simulink model "Casc_Filter_reva"  (Simulink 6.6)
settings: Solver=ode45  StartTime=0.0  StopTime=32768/sampling_freq  RelTol=1e-3
values from neighbouring files (symbols this model uses):
  filter_clk = sampling_freq*clk_mult    (= 375000000)    [Cascade_Taps_reva.m]    (also in Casecade_Taps.m)
  h_g = round(h_g*2^17)/2^17    [Cascade_Taps_reva.m]    (also in Casecade_Taps.m)
  h_k = round(h_k*2^17)/2^17    [Cascade_Taps_reva.m]    (also in Casecade_Taps.m)
  sampling_freq = 125e6    (= 125000000)    [Cascade_Taps_reva.m]    (also in Casecade_Taps.m)
undefined symbols (not defined in the file or in its folder): A, B, Fs, get, PCIN
libraries: xbsIndex_r4 x314, dspsnks4 x3, dspsrcs4 x2, simulink x2
(part 2 of 3)

== system Casc_Filter_reva/DDC/DDC A/Polyphase Kaiser FIR Filter/MAC0 ==
  Count : Inport
  Data In : Inport  Port=2
  Symm Data : Inport  Port=3
  Coeff : Inport  Port=4
  Count Inv : Inport  Port=5
  ASR : xbsIndex_r4/Addressable Shift Register  infer_latency=off  depth=8  initVector=[0]  en=off  dbl_ovrd=off  use_behavioral_HDL=off  use_rpm=off  block_type=addrsr
      settings: block_version=8.2
      settings: infoedit=|
      | Delay of  configurable length.  Any element  in the delay
      |     line   can    be   addressed   and   driven    onto   the   output
      |     port.<P><P>Hardware  notes: Implemented  using SRL16s.
      |     If Virtex-4, Virtex-II or Spartan-3 devices are used, multiple SRLC16s are cascaded together.
  ASR1 : xbsIndex_r4/Addressable Shift Register  infer_latency=off  depth=8  initVector=[0]  en=off  dbl_ovrd=off  use_behavioral_HDL=off  use_rpm=off  block_type=addrsr
      settings: block_version=8.2
      settings: infoedit=|
      | Delay of  configurable length.  Any element  in the delay
      |     line   can    be   addressed   and   driven    onto   the   output
      |     port.<P><P>Hardware  notes: Implemented  using SRL16s.
      |     If Virtex-4, Virtex-II or Spartan-3 devices are used, multiple SRLC16s are cascaded together.
  AddSub1 : xbsIndex_r4/AddSub  mode=Subtraction  use_carryin=off  use_carryout=off  en=off  latency=1  precision=User Defined  arith_type="Signed  (2's comp)"  n_bits=18  bin_pt=16  quantization="Round  (unbiased: +/- Inf)"  overflow=Saturate  dbl_ovrd=off  use_behavioral_HDL=off  pipelined=on  use_rpm=on  block_type=addsub
      settings: block_version=8.2
  Constant4 : xbsIndex_r4/Constant  arith_type=DSP48 Instruction  const=5  n_bits=7  bin_pt=0  explicit_period=off  period=1  equ=P=+(A*B)  opselect=A * B  inp2=PCIN>>17  opr=+  inp1=P  carry=CIN  dbl_ovrd=off  block_type=constant
      settings: block_version=VER_STRING_GOES_HERE
  DSP1 : xbsIndex_r4/DSP48  use_b=Direct from B Port  use_op=on  use_creg=off  use_pcin=off  use_pcout=on  use_bcout=off  rst_all=off  en_all=off  pipeline_a=1  pipeline_b=1  pipeline_c=on  pipeline_p=on  pipeline_mult=on  pipeline_opmode=off  pipeline_sub=off  pipeline_carryin=off  pipeline_carryinsel=off  rst_a=off  rst_b=off  rst_c=off  rst_mult=off  rst_p=off  rst_carry_in=off  rst_ctrl=off  en_a=off  en_b=off  en_c=off  en_mult=off  en_p=off  en_carry_in=off  en_ctrl=off  dbl_ovrd=off  use_synth_model=off  xl_useadderonly=off  block_type=dsp48
      settings: block_version=8.2
  Delay : xbsIndex_r4/Delay  en=off  latency=2  dbl_ovrd=off  reg_retiming=off  block_type=delay
      settings: infoedit=Hardware notes: A delay line is a chain, each link of which is an SRL16 followed by a flip-flop. If register retiming is enabled, the delay line is a chain of flip-flops.  block_version=8.2
  Delay3 : xbsIndex_r4/Delay  en=off  latency=8  dbl_ovrd=off  reg_retiming=off  block_type=delay
      settings: infoedit=Hardware notes: A delay line is a chain, each link of which is an SRL16 followed by a flip-flop. If register retiming is enabled, the delay line is a chain of flip-flops.  block_version=8.2
  Register : xbsIndex_r4/Register  init=0  rst=off  en=off  dbl_ovrd=off  block_type=register
      settings: block_version=8.2
  Register1 : xbsIndex_r4/Register  init=0  rst=off  en=off  dbl_ovrd=off  block_type=register
      settings: block_version=8.2
  Reinterpret : xbsIndex_r4/Reinterpret  force_arith_type=on  arith_type="Signed  (2's comp)"  force_bin_pt=on  bin_pt=0  block_type=cast
      settings: infoedit="Changes type of samples without altering their binary representation.<P><P>Hardware notes: In hardware this block costs nothing.<P><P>Example:  Suppose the input is 6 bits wide, signed, with 2 fractional bits, and the output is forced to unsigned with 0 fractional bits.  Then an input of -2.0 (1110.00 in binary 2's complement) becomes an output of 56 (111000 in binary)."  block_version=VER_STRING_GOES_HERE
  Reinterpret1 : xbsIndex_r4/Reinterpret  force_arith_type=on  arith_type="Signed  (2's comp)"  force_bin_pt=on  bin_pt=0  block_type=cast
      settings: infoedit="Changes type of samples without altering their binary representation.<P><P>Hardware notes: In hardware this block costs nothing.<P><P>Example:  Suppose the input is 6 bits wide, signed, with 2 fractional bits, and the output is forced to unsigned with 0 fractional bits.  Then an input of -2.0 (1110.00 in binary 2's complement) becomes an output of 56 (111000 in binary)."  block_version=VER_STRING_GOES_HERE
  Terminator : Terminator
  Out : Outport
  wires:
  Count/1 -> ASR/2
  Data In/1 -> ASR/1
  ASR/1 -> Register/1
  AddSub1/1 -> Reinterpret/1
  Coeff/1 -> Delay/1
  Delay/1 -> Reinterpret1/1
  Register/1 -> AddSub1/2
  Symm Data/1 -> Delay3/1
  Count Inv/1 -> ASR1/2
  Delay3/1 -> ASR1/1
  ASR1/1 -> Register1/1
  Register1/1 -> AddSub1/1
  Reinterpret/1 -> DSP1/1
  Reinterpret1/1 -> DSP1/2
  Constant4/1 -> DSP1/3
  DSP1/2 -> Out/1
  DSP1/1 -> Terminator/1

== system Casc_Filter_reva/DDC/DDC A/Polyphase Kaiser FIR Filter/MAC1 ==
  Count : Inport
  Data In : Inport  Port=2
  Symm Data : Inport  Port=3
  Coeff : Inport  Port=4
  Count Inv : Inport  Port=5
  ASR : xbsIndex_r4/Addressable Shift Register  infer_latency=off  depth=8  initVector=[0]  en=off  dbl_ovrd=off  use_behavioral_HDL=off  use_rpm=off  block_type=addrsr
      settings: block_version=8.2
      settings: infoedit=|
      | Delay of  configurable length.  Any element  in the delay
      |     line   can    be   addressed   and   driven    onto   the   output
      |     port.<P><P>Hardware  notes: Implemented  using SRL16s.
      |     If Virtex-4, Virtex-II or Spartan-3 devices are used, multiple SRLC16s are cascaded together.
  ASR1 : xbsIndex_r4/Addressable Shift Register  infer_latency=off  depth=8  initVector=[0]  en=off  dbl_ovrd=off  use_behavioral_HDL=off  use_rpm=off  block_type=addrsr
      settings: block_version=8.2
      settings: infoedit=|
      | Delay of  configurable length.  Any element  in the delay
      |     line   can    be   addressed   and   driven    onto   the   output
      |     port.<P><P>Hardware  notes: Implemented  using SRL16s.
      |     If Virtex-4, Virtex-II or Spartan-3 devices are used, multiple SRLC16s are cascaded together.
  AddSub1 : xbsIndex_r4/AddSub  mode=Addition  use_carryin=off  use_carryout=off  en=off  latency=1  precision=User Defined  arith_type="Signed  (2's comp)"  n_bits=18  bin_pt=16  quantization="Round  (unbiased: +/- Inf)"  overflow=Saturate  dbl_ovrd=off  use_behavioral_HDL=off  pipelined=on  use_rpm=on  block_type=addsub
      settings: block_version=8.2
  Constant3 : xbsIndex_r4/Constant  arith_type=DSP48 Instruction  const=5  n_bits=7  bin_pt=0  explicit_period=off  period=1  equ=P=-(A*B)  opselect=Custom  inp2=0  opr=-  inp1=A*B  carry=0  dbl_ovrd=off  block_type=constant
      settings: block_version=VER_STRING_GOES_HERE
  DSP48 : xbsIndex_r4/DSP48  use_b=Direct from B Port  use_op=on  use_creg=off  use_pcin=off  use_pcout=on  use_bcout=off  rst_all=off  en_all=off  pipeline_a=1  pipeline_b=1  pipeline_c=on  pipeline_p=on  pipeline_mult=on  pipeline_opmode=off  pipeline_sub=off  pipeline_carryin=off  pipeline_carryinsel=off  rst_a=off  rst_b=off  rst_c=off  rst_mult=off  rst_p=off  rst_carry_in=off  rst_ctrl=off  en_a=off  en_b=off  en_c=off  en_mult=off  en_p=off  en_carry_in=off  en_ctrl=off  dbl_ovrd=off  use_synth_model=off  xl_useadderonly=off  block_type=dsp48
      settings: block_version=8.2
  Delay : xbsIndex_r4/Delay  en=off  latency=2  dbl_ovrd=off  reg_retiming=off  block_type=delay
      settings: infoedit=Hardware notes: A delay line is a chain, each link of which is an SRL16 followed by a flip-flop. If register retiming is enabled, the delay line is a chain of flip-flops.  block_version=8.2
  Delay3 : xbsIndex_r4/Delay  en=off  latency=8  dbl_ovrd=off  reg_retiming=off  block_type=delay
      settings: infoedit=Hardware notes: A delay line is a chain, each link of which is an SRL16 followed by a flip-flop. If register retiming is enabled, the delay line is a chain of flip-flops.  block_version=8.2
  Register : xbsIndex_r4/Register  init=0  rst=off  en=off  dbl_ovrd=off  block_type=register
      settings: block_version=8.2
  Register1 : xbsIndex_r4/Register  init=0  rst=off  en=off  dbl_ovrd=off  block_type=register
      settings: block_version=8.2
  Reinterpret : xbsIndex_r4/Reinterpret  force_arith_type=on  arith_type="Signed  (2's comp)"  force_bin_pt=on  bin_pt=0  block_type=cast
      settings: infoedit="Changes type of samples without altering their binary representation.<P><P>Hardware notes: In hardware this block costs nothing.<P><P>Example:  Suppose the input is 6 bits wide, signed, with 2 fractional bits, and the output is forced to unsigned with 0 fractional bits.  Then an input of -2.0 (1110.00 in binary 2's complement) becomes an output of 56 (111000 in binary)."  block_version=VER_STRING_GOES_HERE
  Reinterpret1 : xbsIndex_r4/Reinterpret  force_arith_type=on  arith_type="Signed  (2's comp)"  force_bin_pt=on  bin_pt=0  block_type=cast
      settings: infoedit="Changes type of samples without altering their binary representation.<P><P>Hardware notes: In hardware this block costs nothing.<P><P>Example:  Suppose the input is 6 bits wide, signed, with 2 fractional bits, and the output is forced to unsigned with 0 fractional bits.  Then an input of -2.0 (1110.00 in binary 2's complement) becomes an output of 56 (111000 in binary)."  block_version=VER_STRING_GOES_HERE
  Terminator : Terminator
  Out : Outport
  wires:
  Count/1 -> ASR/2
  Data In/1 -> ASR/1
  AddSub1/1 -> Reinterpret/1
  Coeff/1 -> Delay/1
  DSP48/2 -> Out/1
  Delay/1 -> Reinterpret1/1
  ASR/1 -> Register/1
  Register/1 -> AddSub1/1
  Symm Data/1 -> Delay3/1
  Count Inv/1 -> ASR1/2
  Delay3/1 -> ASR1/1
  ASR1/1 -> Register1/1
  Register1/1 -> AddSub1/2
  Reinterpret/1 -> DSP48/1
  Reinterpret1/1 -> DSP48/2
  Constant3/1 -> DSP48/3
  DSP48/1 -> Terminator/1

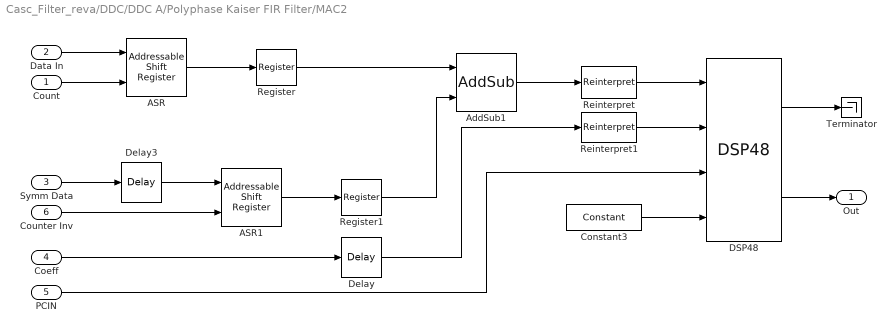
== system Casc_Filter_reva/DDC/DDC A/Polyphase Kaiser FIR Filter/MAC2 ==
  Count : Inport
  Data In : Inport  Port=2
  Symm Data : Inport  Port=3
  Coeff : Inport  Port=4
  PCIN : Inport  Port=5
  Counter Inv : Inport  Port=6
  ASR : xbsIndex_r4/Addressable Shift Register  infer_latency=off  depth=8  initVector=[0]  en=off  dbl_ovrd=off  use_behavioral_HDL=off  use_rpm=off  block_type=addrsr
      settings: block_version=8.2
      settings: infoedit=|
      | Delay of  configurable length.  Any element  in the delay
      |     line   can    be   addressed   and   driven    onto   the   output
      |     port.<P><P>Hardware  notes: Implemented  using SRL16s.
      |     If Virtex-4, Virtex-II or Spartan-3 devices are used, multiple SRLC16s are cascaded together.
  ASR1 : xbsIndex_r4/Addressable Shift Register  infer_latency=off  depth=8  initVector=[0]  en=off  dbl_ovrd=off  use_behavioral_HDL=off  use_rpm=off  block_type=addrsr
      settings: block_version=8.2
      settings: infoedit=|
      | Delay of  configurable length.  Any element  in the delay
      |     line   can    be   addressed   and   driven    onto   the   output
      |     port.<P><P>Hardware  notes: Implemented  using SRL16s.
      |     If Virtex-4, Virtex-II or Spartan-3 devices are used, multiple SRLC16s are cascaded together.
  AddSub1 : xbsIndex_r4/AddSub  mode=Subtraction  use_carryin=off  use_carryout=off  en=off  latency=1  precision=User Defined  arith_type="Signed  (2's comp)"  n_bits=18  bin_pt=16  quantization="Round  (unbiased: +/- Inf)"  overflow=Saturate  dbl_ovrd=off  use_behavioral_HDL=off  pipelined=on  use_rpm=on  block_type=addsub
      settings: block_version=8.2
  Constant3 : xbsIndex_r4/Constant  arith_type=DSP48 Instruction  const=53  n_bits=7  bin_pt=0  explicit_period=off  period=1  equ=P=PCIN+(A*B)  opselect=PCIN + A*B  inp2=PCIN>>17  opr=+  inp1=P  carry=CIN  dbl_ovrd=off  block_type=constant
      settings: block_version=VER_STRING_GOES_HERE
  DSP48 : xbsIndex_r4/DSP48  use_b=Direct from B Port  use_op=on  use_creg=off  use_pcin=on  use_pcout=on  use_bcout=off  rst_all=off  en_all=off  pipeline_a=2  pipeline_b=2  pipeline_c=on  pipeline_p=on  pipeline_mult=on  pipeline_opmode=off  pipeline_sub=off  pipeline_carryin=off  pipeline_carryinsel=off  rst_a=off  rst_b=off  rst_c=off  rst_mult=off  rst_p=off  rst_carry_in=off  rst_ctrl=off  en_a=off  en_b=off  en_c=off  en_mult=off  en_p=off  en_carry_in=off  en_ctrl=off  dbl_ovrd=off  use_synth_model=off  xl_useadderonly=off  block_type=dsp48
      settings: block_version=8.2
  Delay : xbsIndex_r4/Delay  en=off  latency=2  dbl_ovrd=off  reg_retiming=off  block_type=delay
      settings: infoedit=Hardware notes: A delay line is a chain, each link of which is an SRL16 followed by a flip-flop. If register retiming is enabled, the delay line is a chain of flip-flops.  block_version=8.2
  Delay3 : xbsIndex_r4/Delay  en=off  latency=8  dbl_ovrd=off  reg_retiming=off  block_type=delay
      settings: infoedit=Hardware notes: A delay line is a chain, each link of which is an SRL16 followed by a flip-flop. If register retiming is enabled, the delay line is a chain of flip-flops.  block_version=8.2
  Register : xbsIndex_r4/Register  init=0  rst=off  en=off  dbl_ovrd=off  block_type=register
      settings: block_version=8.2
  Register1 : xbsIndex_r4/Register  init=0  rst=off  en=off  dbl_ovrd=off  block_type=register
      settings: block_version=8.2
  Reinterpret : xbsIndex_r4/Reinterpret  force_arith_type=on  arith_type="Signed  (2's comp)"  force_bin_pt=on  bin_pt=0  block_type=cast
      settings: infoedit="Changes type of samples without altering their binary representation.<P><P>Hardware notes: In hardware this block costs nothing.<P><P>Example:  Suppose the input is 6 bits wide, signed, with 2 fractional bits, and the output is forced to unsigned with 0 fractional bits.  Then an input of -2.0 (1110.00 in binary 2's complement) becomes an output of 56 (111000 in binary)."  block_version=VER_STRING_GOES_HERE
  Reinterpret1 : xbsIndex_r4/Reinterpret  force_arith_type=on  arith_type="Signed  (2's comp)"  force_bin_pt=on  bin_pt=0  block_type=cast
      settings: infoedit="Changes type of samples without altering their binary representation.<P><P>Hardware notes: In hardware this block costs nothing.<P><P>Example:  Suppose the input is 6 bits wide, signed, with 2 fractional bits, and the output is forced to unsigned with 0 fractional bits.  Then an input of -2.0 (1110.00 in binary 2's complement) becomes an output of 56 (111000 in binary)."  block_version=VER_STRING_GOES_HERE
  Terminator : Terminator
  Out : Outport
  wires:
  Count/1 -> ASR/2
  Data In/1 -> ASR/1
  AddSub1/1 -> Reinterpret/1
  Coeff/1 -> Delay/1
  Delay/1 -> Reinterpret1/1
  ASR/1 -> Register/1
  PCIN/1 -> DSP48/3
  Register/1 -> AddSub1/1
  Symm Data/1 -> Delay3/1
  Counter Inv/1 -> ASR1/2
  Delay3/1 -> ASR1/1
  ASR1/1 -> Register1/1
  Register1/1 -> AddSub1/2
  Reinterpret/1 -> DSP48/1
  Reinterpret1/1 -> DSP48/2
  Constant3/1 -> DSP48/4
  DSP48/1 -> Terminator/1
  DSP48/2 -> Out/1

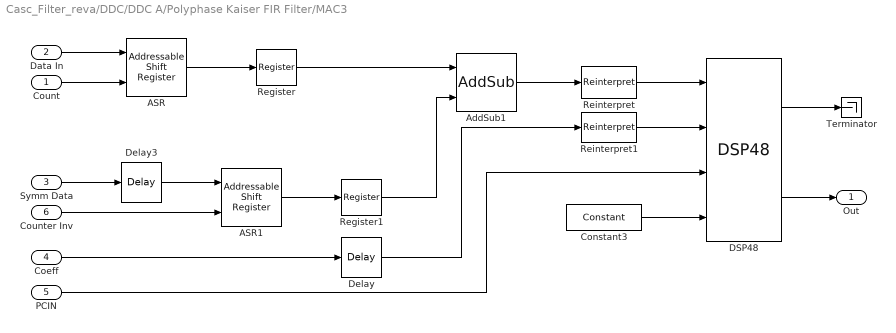
== system Casc_Filter_reva/DDC/DDC A/Polyphase Kaiser FIR Filter/MAC3 ==
  Count : Inport
  Data In : Inport  Port=2
  Symm Data : Inport  Port=3
  Coeff : Inport  Port=4
  PCIN : Inport  Port=5
  Counter Inv : Inport  Port=6
  ASR : xbsIndex_r4/Addressable Shift Register  infer_latency=off  depth=8  initVector=[0]  en=off  dbl_ovrd=off  use_behavioral_HDL=off  use_rpm=off  block_type=addrsr
      settings: block_version=8.2
      settings: infoedit=|
      | Delay of  configurable length.  Any element  in the delay
      |     line   can    be   addressed   and   driven    onto   the   output
      |     port.<P><P>Hardware  notes: Implemented  using SRL16s.
      |     If Virtex-4, Virtex-II or Spartan-3 devices are used, multiple SRLC16s are cascaded together.
  ASR1 : xbsIndex_r4/Addressable Shift Register  infer_latency=off  depth=8  initVector=[0]  en=off  dbl_ovrd=off  use_behavioral_HDL=off  use_rpm=off  block_type=addrsr
      settings: block_version=8.2
      settings: infoedit=|
      | Delay of  configurable length.  Any element  in the delay
      |     line   can    be   addressed   and   driven    onto   the   output
      |     port.<P><P>Hardware  notes: Implemented  using SRL16s.
      |     If Virtex-4, Virtex-II or Spartan-3 devices are used, multiple SRLC16s are cascaded together.
  AddSub1 : xbsIndex_r4/AddSub  mode=Addition  use_carryin=off  use_carryout=off  en=off  latency=1  precision=User Defined  arith_type="Signed  (2's comp)"  n_bits=18  bin_pt=16  quantization="Round  (unbiased: +/- Inf)"  overflow=Saturate  dbl_ovrd=off  use_behavioral_HDL=off  pipelined=on  use_rpm=on  block_type=addsub
      settings: block_version=8.2
  Constant3 : xbsIndex_r4/Constant  arith_type=DSP48 Instruction  const=53  n_bits=7  bin_pt=0  explicit_period=off  period=1  equ=P=PCIN+(A*B)  opselect=Custom  inp2=PCIN  opr=+  inp1=A*B  carry=0  dbl_ovrd=off  block_type=constant
      settings: block_version=VER_STRING_GOES_HERE
  DSP48 : xbsIndex_r4/DSP48  use_b=Direct from B Port  use_op=on  use_creg=off  use_pcin=on  use_pcout=on  use_bcout=off  rst_all=off  en_all=off  pipeline_a=2  pipeline_b=2  pipeline_c=on  pipeline_p=on  pipeline_mult=on  pipeline_opmode=off  pipeline_sub=off  pipeline_carryin=off  pipeline_carryinsel=off  rst_a=off  rst_b=off  rst_c=off  rst_mult=off  rst_p=off  rst_carry_in=off  rst_ctrl=off  en_a=off  en_b=off  en_c=off  en_mult=off  en_p=off  en_carry_in=off  en_ctrl=off  dbl_ovrd=off  use_synth_model=off  xl_useadderonly=off  block_type=dsp48
      settings: block_version=8.2
  Delay : xbsIndex_r4/Delay  en=off  latency=2  dbl_ovrd=off  reg_retiming=off  block_type=delay
      settings: infoedit=Hardware notes: A delay line is a chain, each link of which is an SRL16 followed by a flip-flop. If register retiming is enabled, the delay line is a chain of flip-flops.  block_version=8.2
  Delay3 : xbsIndex_r4/Delay  en=off  latency=8  dbl_ovrd=off  reg_retiming=off  block_type=delay
      settings: infoedit=Hardware notes: A delay line is a chain, each link of which is an SRL16 followed by a flip-flop. If register retiming is enabled, the delay line is a chain of flip-flops.  block_version=8.2
  Register : xbsIndex_r4/Register  init=0  rst=off  en=off  dbl_ovrd=off  block_type=register
      settings: block_version=8.2
  Register1 : xbsIndex_r4/Register  init=0  rst=off  en=off  dbl_ovrd=off  block_type=register
      settings: block_version=8.2
  Reinterpret : xbsIndex_r4/Reinterpret  force_arith_type=on  arith_type="Signed  (2's comp)"  force_bin_pt=on  bin_pt=0  block_type=cast
      settings: infoedit="Changes type of samples without altering their binary representation.<P><P>Hardware notes: In hardware this block costs nothing.<P><P>Example:  Suppose the input is 6 bits wide, signed, with 2 fractional bits, and the output is forced to unsigned with 0 fractional bits.  Then an input of -2.0 (1110.00 in binary 2's complement) becomes an output of 56 (111000 in binary)."  block_version=VER_STRING_GOES_HERE
  Reinterpret1 : xbsIndex_r4/Reinterpret  force_arith_type=on  arith_type="Signed  (2's comp)"  force_bin_pt=on  bin_pt=0  block_type=cast
      settings: infoedit="Changes type of samples without altering their binary representation.<P><P>Hardware notes: In hardware this block costs nothing.<P><P>Example:  Suppose the input is 6 bits wide, signed, with 2 fractional bits, and the output is forced to unsigned with 0 fractional bits.  Then an input of -2.0 (1110.00 in binary 2's complement) becomes an output of 56 (111000 in binary)."  block_version=VER_STRING_GOES_HERE
  Terminator : Terminator
  Out : Outport
  wires:
  Count/1 -> ASR/2
  Data In/1 -> ASR/1
  AddSub1/1 -> Reinterpret/1
  Coeff/1 -> Delay/1
  Delay/1 -> Reinterpret1/1
  ASR/1 -> Register/1
  PCIN/1 -> DSP48/3
  Register/1 -> AddSub1/1
  Symm Data/1 -> Delay3/1
  Counter Inv/1 -> ASR1/2
  Delay3/1 -> ASR1/1
  ASR1/1 -> Register1/1
  Register1/1 -> AddSub1/2
  Reinterpret/1 -> DSP48/1
  Reinterpret1/1 -> DSP48/2
  Constant3/1 -> DSP48/4
  DSP48/1 -> Terminator/1
  DSP48/2 -> Out/1

== system Casc_Filter_reva/DDC/DDC A/Polyphase Kaiser FIR Filter/MAC4 ==
  Count : Inport
  Data In : Inport  Port=2
  Symm Data : Inport  Port=3
  Coeff : Inport  Port=4
  PCIN : Inport  Port=5
  Counter Inv : Inport  Port=6
  ASR : xbsIndex_r4/Addressable Shift Register  infer_latency=off  depth=8  initVector=[0]  en=off  dbl_ovrd=off  use_behavioral_HDL=off  use_rpm=off  block_type=addrsr
      settings: block_version=8.2
      settings: infoedit=|
      | Delay of  configurable length.  Any element  in the delay
      |     line   can    be   addressed   and   driven    onto   the   output
      |     port.<P><P>Hardware  notes: Implemented  using SRL16s.
      |     If Virtex-4, Virtex-II or Spartan-3 devices are used, multiple SRLC16s are cascaded together.
  ASR1 : xbsIndex_r4/Addressable Shift Register  infer_latency=off  depth=8  initVector=[0]  en=off  dbl_ovrd=off  use_behavioral_HDL=off  use_rpm=off  block_type=addrsr
      settings: block_version=8.2
      settings: infoedit=|
      | Delay of  configurable length.  Any element  in the delay
      |     line   can    be   addressed   and   driven    onto   the   output
      |     port.<P><P>Hardware  notes: Implemented  using SRL16s.
      |     If Virtex-4, Virtex-II or Spartan-3 devices are used, multiple SRLC16s are cascaded together.
  AddSub1 : xbsIndex_r4/AddSub  mode=Subtraction  use_carryin=off  use_carryout=off  en=off  latency=1  precision=User Defined  arith_type="Signed  (2's comp)"  n_bits=18  bin_pt=16  quantization="Round  (unbiased: +/- Inf)"  overflow=Saturate  dbl_ovrd=off  use_behavioral_HDL=off  pipelined=on  use_rpm=on  block_type=addsub
      settings: block_version=8.2
  Constant3 : xbsIndex_r4/Constant  arith_type=DSP48 Instruction  const=53  n_bits=7  bin_pt=0  explicit_period=off  period=1  equ=P=PCIN+(A*B)  opselect=PCIN + A*B  inp2=PCIN>>17  opr=+  inp1=P  carry=CIN  dbl_ovrd=off  block_type=constant
      settings: block_version=VER_STRING_GOES_HERE
  DSP48 : xbsIndex_r4/DSP48  use_b=Direct from B Port  use_op=on  use_creg=off  use_pcin=on  use_pcout=on  use_bcout=off  rst_all=off  en_all=off  pipeline_a=2  pipeline_b=2  pipeline_c=on  pipeline_p=on  pipeline_mult=on  pipeline_opmode=off  pipeline_sub=off  pipeline_carryin=off  pipeline_carryinsel=off  rst_a=off  rst_b=off  rst_c=off  rst_mult=off  rst_p=off  rst_carry_in=off  rst_ctrl=off  en_a=off  en_b=off  en_c=off  en_mult=off  en_p=off  en_carry_in=off  en_ctrl=off  dbl_ovrd=off  use_synth_model=off  xl_useadderonly=off  block_type=dsp48
      settings: block_version=8.2
  Delay : xbsIndex_r4/Delay  en=off  latency=2  dbl_ovrd=off  reg_retiming=off  block_type=delay
      settings: infoedit=Hardware notes: A delay line is a chain, each link of which is an SRL16 followed by a flip-flop. If register retiming is enabled, the delay line is a chain of flip-flops.  block_version=8.2
  Delay3 : xbsIndex_r4/Delay  en=off  latency=8  dbl_ovrd=off  reg_retiming=off  block_type=delay
      settings: infoedit=Hardware notes: A delay line is a chain, each link of which is an SRL16 followed by a flip-flop. If register retiming is enabled, the delay line is a chain of flip-flops.  block_version=8.2
  Register : xbsIndex_r4/Register  init=0  rst=off  en=off  dbl_ovrd=off  block_type=register
      settings: block_version=8.2
  Register1 : xbsIndex_r4/Register  init=0  rst=off  en=off  dbl_ovrd=off  block_type=register
      settings: block_version=8.2
  Reinterpret : xbsIndex_r4/Reinterpret  force_arith_type=on  arith_type="Signed  (2's comp)"  force_bin_pt=on  bin_pt=0  block_type=cast
      settings: infoedit="Changes type of samples without altering their binary representation.<P><P>Hardware notes: In hardware this block costs nothing.<P><P>Example:  Suppose the input is 6 bits wide, signed, with 2 fractional bits, and the output is forced to unsigned with 0 fractional bits.  Then an input of -2.0 (1110.00 in binary 2's complement) becomes an output of 56 (111000 in binary)."  block_version=VER_STRING_GOES_HERE
  Reinterpret1 : xbsIndex_r4/Reinterpret  force_arith_type=on  arith_type="Signed  (2's comp)"  force_bin_pt=on  bin_pt=0  block_type=cast
      settings: infoedit="Changes type of samples without altering their binary representation.<P><P>Hardware notes: In hardware this block costs nothing.<P><P>Example:  Suppose the input is 6 bits wide, signed, with 2 fractional bits, and the output is forced to unsigned with 0 fractional bits.  Then an input of -2.0 (1110.00 in binary 2's complement) becomes an output of 56 (111000 in binary)."  block_version=VER_STRING_GOES_HERE
  Terminator : Terminator
  Out : Outport
  wires:
  Count/1 -> ASR/2
  Data In/1 -> ASR/1
  AddSub1/1 -> Reinterpret/1
  Coeff/1 -> Delay/1
  Delay/1 -> Reinterpret1/1
  ASR/1 -> Register/1
  PCIN/1 -> DSP48/3
  Register/1 -> AddSub1/2
  Symm Data/1 -> Delay3/1
  Counter Inv/1 -> ASR1/2
  Delay3/1 -> ASR1/1
  ASR1/1 -> Register1/1
  Reinterpret/1 -> DSP48/1
  Reinterpret1/1 -> DSP48/2
  Constant3/1 -> DSP48/4
  DSP48/1 -> Terminator/1
  DSP48/2 -> Out/1
  Register1/1 -> AddSub1/1

== system Casc_Filter_reva/DDC/DDC A/Polyphase Kaiser FIR Filter/MAC5 ==
  Count : Inport
  Data In : Inport  Port=2
  Symm Data : Inport  Port=3
  Coeff : Inport  Port=4
  PCIN : Inport  Port=5
  Counter Inv : Inport  Port=6
  ASR : xbsIndex_r4/Addressable Shift Register  infer_latency=off  depth=8  initVector=[0]  en=off  dbl_ovrd=off  use_behavioral_HDL=off  use_rpm=off  block_type=addrsr
      settings: block_version=8.2
      settings: infoedit=|
      | Delay of  configurable length.  Any element  in the delay
      |     line   can    be   addressed   and   driven    onto   the   output
      |     port.<P><P>Hardware  notes: Implemented  using SRL16s.
      |     If Virtex-4, Virtex-II or Spartan-3 devices are used, multiple SRLC16s are cascaded together.
  ASR1 : xbsIndex_r4/Addressable Shift Register  infer_latency=off  depth=8  initVector=[0]  en=off  dbl_ovrd=off  use_behavioral_HDL=off  use_rpm=off  block_type=addrsr
      settings: block_version=8.2
      settings: infoedit=|
      | Delay of  configurable length.  Any element  in the delay
      |     line   can    be   addressed   and   driven    onto   the   output
      |     port.<P><P>Hardware  notes: Implemented  using SRL16s.
      |     If Virtex-4, Virtex-II or Spartan-3 devices are used, multiple SRLC16s are cascaded together.
  AddSub1 : xbsIndex_r4/AddSub  mode=Addition  use_carryin=off  use_carryout=off  en=off  latency=1  precision=User Defined  arith_type="Signed  (2's comp)"  n_bits=18  bin_pt=16  quantization="Round  (unbiased: +/- Inf)"  overflow=Saturate  dbl_ovrd=off  use_behavioral_HDL=off  pipelined=on  use_rpm=on  block_type=addsub
      settings: block_version=8.2
  Constant3 : xbsIndex_r4/Constant  arith_type=DSP48 Instruction  const=53  n_bits=7  bin_pt=0  explicit_period=off  period=1  equ=P=PCIN-(A*B)  opselect=Custom  inp2=PCIN  opr=-  inp1=A*B  carry=0  dbl_ovrd=off  block_type=constant
      settings: block_version=VER_STRING_GOES_HERE
  DSP48 : xbsIndex_r4/DSP48  use_b=Direct from B Port  use_op=on  use_creg=off  use_pcin=on  use_pcout=on  use_bcout=off  rst_all=off  en_all=off  pipeline_a=2  pipeline_b=2  pipeline_c=on  pipeline_p=on  pipeline_mult=on  pipeline_opmode=off  pipeline_sub=off  pipeline_carryin=off  pipeline_carryinsel=off  rst_a=off  rst_b=off  rst_c=off  rst_mult=off  rst_p=off  rst_carry_in=off  rst_ctrl=off  en_a=off  en_b=off  en_c=off  en_mult=off  en_p=off  en_carry_in=off  en_ctrl=off  dbl_ovrd=off  use_synth_model=off  xl_useadderonly=off  block_type=dsp48
      settings: block_version=8.2
  Delay : xbsIndex_r4/Delay  en=off  latency=2  dbl_ovrd=off  reg_retiming=off  block_type=delay
      settings: infoedit=Hardware notes: A delay line is a chain, each link of which is an SRL16 followed by a flip-flop. If register retiming is enabled, the delay line is a chain of flip-flops.  block_version=8.2
  Delay3 : xbsIndex_r4/Delay  en=off  latency=8  dbl_ovrd=off  reg_retiming=off  block_type=delay
      settings: infoedit=Hardware notes: A delay line is a chain, each link of which is an SRL16 followed by a flip-flop. If register retiming is enabled, the delay line is a chain of flip-flops.  block_version=8.2
  Register : xbsIndex_r4/Register  init=0  rst=off  en=off  dbl_ovrd=off  block_type=register
      settings: block_version=8.2
  Register1 : xbsIndex_r4/Register  init=0  rst=off  en=off  dbl_ovrd=off  block_type=register
      settings: block_version=8.2
  Reinterpret : xbsIndex_r4/Reinterpret  force_arith_type=on  arith_type="Signed  (2's comp)"  force_bin_pt=on  bin_pt=0  block_type=cast
      settings: infoedit="Changes type of samples without altering their binary representation.<P><P>Hardware notes: In hardware this block costs nothing.<P><P>Example:  Suppose the input is 6 bits wide, signed, with 2 fractional bits, and the output is forced to unsigned with 0 fractional bits.  Then an input of -2.0 (1110.00 in binary 2's complement) becomes an output of 56 (111000 in binary)."  block_version=VER_STRING_GOES_HERE
  Reinterpret1 : xbsIndex_r4/Reinterpret  force_arith_type=on  arith_type="Signed  (2's comp)"  force_bin_pt=on  bin_pt=0  block_type=cast
      settings: infoedit="Changes type of samples without altering their binary representation.<P><P>Hardware notes: In hardware this block costs nothing.<P><P>Example:  Suppose the input is 6 bits wide, signed, with 2 fractional bits, and the output is forced to unsigned with 0 fractional bits.  Then an input of -2.0 (1110.00 in binary 2's complement) becomes an output of 56 (111000 in binary)."  block_version=VER_STRING_GOES_HERE
  Terminator : Terminator
  Out : Outport
  wires:
  Count/1 -> ASR/2
  Data In/1 -> ASR/1
  AddSub1/1 -> Reinterpret/1
  Coeff/1 -> Delay/1
  Delay/1 -> Reinterpret1/1
  ASR/1 -> Register/1
  PCIN/1 -> DSP48/3
  Register/1 -> AddSub1/1
  Symm Data/1 -> Delay3/1
  Counter Inv/1 -> ASR1/2
  Delay3/1 -> ASR1/1
  ASR1/1 -> Register1/1
  Register1/1 -> AddSub1/2
  Reinterpret/1 -> DSP48/1
  Reinterpret1/1 -> DSP48/2
  Constant3/1 -> DSP48/4
  DSP48/1 -> Terminator/1
  DSP48/2 -> Out/1

== system Casc_Filter_reva/DDC/DDC A/Polyphase Kaiser FIR Filter/MAC6 ==
  Count : Inport
  Data In : Inport  Port=2
  Symm Data : Inport  Port=3
  Coeff : Inport  Port=4
  PCIN : Inport  Port=5
  Counter Inv : Inport  Port=6
  ASR : xbsIndex_r4/Addressable Shift Register  infer_latency=off  depth=8  initVector=[0]  en=off  dbl_ovrd=off  use_behavioral_HDL=off  use_rpm=off  block_type=addrsr
      settings: block_version=8.2
      settings: infoedit=|
      | Delay of  configurable length.  Any element  in the delay
      |     line   can    be   addressed   and   driven    onto   the   output
      |     port.<P><P>Hardware  notes: Implemented  using SRL16s.
      |     If Virtex-4, Virtex-II or Spartan-3 devices are used, multiple SRLC16s are cascaded together.
  ASR1 : xbsIndex_r4/Addressable Shift Register  infer_latency=off  depth=8  initVector=[0]  en=off  dbl_ovrd=off  use_behavioral_HDL=off  use_rpm=off  block_type=addrsr
      settings: block_version=8.2
      settings: infoedit=|
      | Delay of  configurable length.  Any element  in the delay
      |     line   can    be   addressed   and   driven    onto   the   output
      |     port.<P><P>Hardware  notes: Implemented  using SRL16s.
      |     If Virtex-4, Virtex-II or Spartan-3 devices are used, multiple SRLC16s are cascaded together.
  AddSub1 : xbsIndex_r4/AddSub  mode=Subtraction  use_carryin=off  use_carryout=off  en=off  latency=1  precision=User Defined  arith_type="Signed  (2's comp)"  n_bits=18  bin_pt=16  quantization="Round  (unbiased: +/- Inf)"  overflow=Saturate  dbl_ovrd=off  use_behavioral_HDL=off  pipelined=on  use_rpm=on  block_type=addsub
      settings: block_version=8.2
  Constant3 : xbsIndex_r4/Constant  arith_type=DSP48 Instruction  const=53  n_bits=7  bin_pt=0  explicit_period=off  period=1  equ=P=PCIN+(A*B)  opselect=PCIN + A*B  inp2=PCIN>>17  opr=+  inp1=P  carry=CIN  dbl_ovrd=off  block_type=constant
      settings: block_version=VER_STRING_GOES_HERE
  DSP48 : xbsIndex_r4/DSP48  use_b=Direct from B Port  use_op=on  use_creg=off  use_pcin=on  use_pcout=on  use_bcout=off  rst_all=off  en_all=off  pipeline_a=2  pipeline_b=2  pipeline_c=on  pipeline_p=on  pipeline_mult=on  pipeline_opmode=off  pipeline_sub=off  pipeline_carryin=off  pipeline_carryinsel=off  rst_a=off  rst_b=off  rst_c=off  rst_mult=off  rst_p=off  rst_carry_in=off  rst_ctrl=off  en_a=off  en_b=off  en_c=off  en_mult=off  en_p=off  en_carry_in=off  en_ctrl=off  dbl_ovrd=off  use_synth_model=off  xl_useadderonly=off  block_type=dsp48
      settings: block_version=8.2
  Delay : xbsIndex_r4/Delay  en=off  latency=2  dbl_ovrd=off  reg_retiming=off  block_type=delay
      settings: infoedit=Hardware notes: A delay line is a chain, each link of which is an SRL16 followed by a flip-flop. If register retiming is enabled, the delay line is a chain of flip-flops.  block_version=8.2
  Delay3 : xbsIndex_r4/Delay  en=off  latency=8  dbl_ovrd=off  reg_retiming=off  block_type=delay
      settings: infoedit=Hardware notes: A delay line is a chain, each link of which is an SRL16 followed by a flip-flop. If register retiming is enabled, the delay line is a chain of flip-flops.  block_version=8.2
  Register : xbsIndex_r4/Register  init=0  rst=off  en=off  dbl_ovrd=off  block_type=register
      settings: block_version=8.2
  Register1 : xbsIndex_r4/Register  init=0  rst=off  en=off  dbl_ovrd=off  block_type=register
      settings: block_version=8.2
  Reinterpret : xbsIndex_r4/Reinterpret  force_arith_type=on  arith_type="Signed  (2's comp)"  force_bin_pt=on  bin_pt=0  block_type=cast
      settings: infoedit="Changes type of samples without altering their binary representation.<P><P>Hardware notes: In hardware this block costs nothing.<P><P>Example:  Suppose the input is 6 bits wide, signed, with 2 fractional bits, and the output is forced to unsigned with 0 fractional bits.  Then an input of -2.0 (1110.00 in binary 2's complement) becomes an output of 56 (111000 in binary)."  block_version=VER_STRING_GOES_HERE
  Reinterpret1 : xbsIndex_r4/Reinterpret  force_arith_type=on  arith_type="Signed  (2's comp)"  force_bin_pt=on  bin_pt=0  block_type=cast
      settings: infoedit="Changes type of samples without altering their binary representation.<P><P>Hardware notes: In hardware this block costs nothing.<P><P>Example:  Suppose the input is 6 bits wide, signed, with 2 fractional bits, and the output is forced to unsigned with 0 fractional bits.  Then an input of -2.0 (1110.00 in binary 2's complement) becomes an output of 56 (111000 in binary)."  block_version=VER_STRING_GOES_HERE
  Terminator : Terminator
  Out : Outport
  wires:
  Count/1 -> ASR/2
  Data In/1 -> ASR/1
  AddSub1/1 -> Reinterpret/1
  Coeff/1 -> Delay/1
  Delay/1 -> Reinterpret1/1
  ASR/1 -> Register/1
  PCIN/1 -> DSP48/3
  Register/1 -> AddSub1/1
  Symm Data/1 -> Delay3/1
  Counter Inv/1 -> ASR1/2
  Delay3/1 -> ASR1/1
  ASR1/1 -> Register1/1
  Register1/1 -> AddSub1/2
  Reinterpret/1 -> DSP48/1
  Reinterpret1/1 -> DSP48/2
  Constant3/1 -> DSP48/4
  DSP48/1 -> Terminator/1
  DSP48/2 -> Out/1

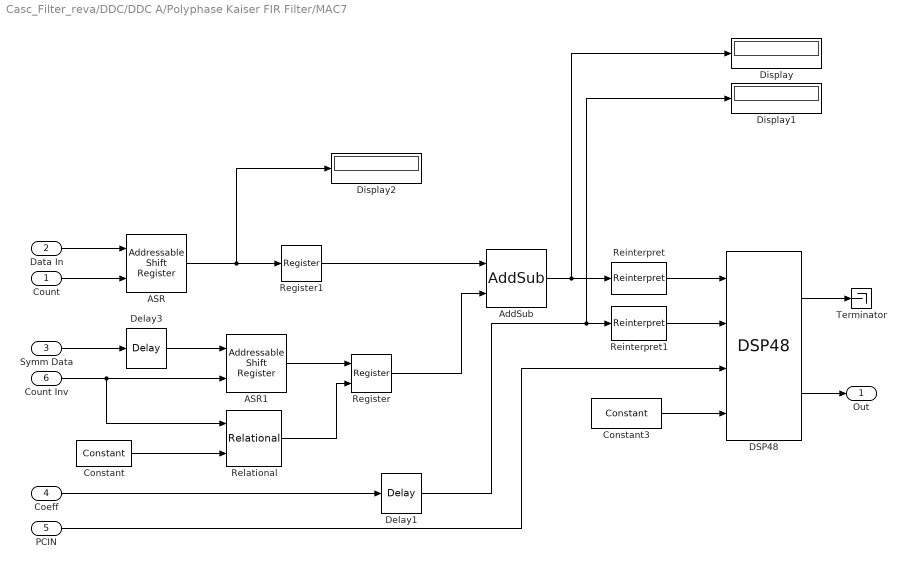
== system Casc_Filter_reva/DDC/DDC A/Polyphase Kaiser FIR Filter/MAC7 ==
  Count : Inport
  Data In : Inport  Port=2
  Symm Data : Inport  Port=3
  Coeff : Inport  Port=4
  PCIN : Inport  Port=5
  Count Inv : Inport  Port=6
  ASR : xbsIndex_r4/Addressable Shift Register  infer_latency=off  depth=8  initVector=[0]  en=off  dbl_ovrd=off  use_behavioral_HDL=off  use_rpm=off  block_type=addrsr
      settings: block_version=8.2
      settings: infoedit=|
      | Delay of  configurable length.  Any element  in the delay
      |     line   can    be   addressed   and   driven    onto   the   output
      |     port.<P><P>Hardware  notes: Implemented  using SRL16s.
      |     If Virtex-4, Virtex-II or Spartan-3 devices are used, multiple SRLC16s are cascaded together.
  ASR1 : xbsIndex_r4/Addressable Shift Register  infer_latency=off  depth=8  initVector=[0]  en=off  dbl_ovrd=off  use_behavioral_HDL=off  use_rpm=off  block_type=addrsr
      settings: block_version=8.2
      settings: infoedit=|
      | Delay of  configurable length.  Any element  in the delay
      |     line   can    be   addressed   and   driven    onto   the   output
      |     port.<P><P>Hardware  notes: Implemented  using SRL16s.
      |     If Virtex-4, Virtex-II or Spartan-3 devices are used, multiple SRLC16s are cascaded together.
  AddSub : xbsIndex_r4/AddSub  mode=Addition  use_carryin=off  use_carryout=off  en=off  latency=1  precision=User Defined  arith_type="Signed  (2's comp)"  n_bits=18  bin_pt=16  quantization="Round  (unbiased: +/- Inf)"  overflow=Saturate  dbl_ovrd=off  use_behavioral_HDL=off  pipelined=on  use_rpm=on  block_type=addsub
      settings: block_version=8.2
  Constant : xbsIndex_r4/Constant  arith_type=Unsigned  const=1  n_bits=4  bin_pt=0  explicit_period=off  period=1  equ=P=C  opselect=C  inp2=PCIN>>17  opr=+  inp1=P  carry=CIN  dbl_ovrd=off  block_type=constant
      settings: block_version=8.2
  Constant3 : xbsIndex_r4/Constant  arith_type=DSP48 Instruction  const=53  n_bits=7  bin_pt=0  explicit_period=off  period=1  equ=P=PCIN+(A*B)  opselect=Custom  inp2=PCIN  opr=+  inp1=A*B  carry=0  dbl_ovrd=off  block_type=constant
      settings: block_version=VER_STRING_GOES_HERE
  DSP48 : xbsIndex_r4/DSP48  use_b=Direct from B Port  use_op=on  use_creg=off  use_pcin=on  use_pcout=on  use_bcout=off  rst_all=off  en_all=off  pipeline_a=2  pipeline_b=2  pipeline_c=on  pipeline_p=on  pipeline_mult=on  pipeline_opmode=off  pipeline_sub=off  pipeline_carryin=off  pipeline_carryinsel=off  rst_a=off  rst_b=off  rst_c=off  rst_mult=off  rst_p=off  rst_carry_in=off  rst_ctrl=off  en_a=off  en_b=off  en_c=off  en_mult=off  en_p=off  en_carry_in=off  en_ctrl=off  dbl_ovrd=off  use_synth_model=off  xl_useadderonly=off  block_type=dsp48
      settings: block_version=8.2
  Delay1 : xbsIndex_r4/Delay  en=off  latency=2  dbl_ovrd=off  reg_retiming=off  block_type=delay
      settings: infoedit=Hardware notes: A delay line is a chain, each link of which is an SRL16 followed by a flip-flop. If register retiming is enabled, the delay line is a chain of flip-flops.  block_version=8.2
  Delay3 : xbsIndex_r4/Delay  en=off  latency=7  dbl_ovrd=off  reg_retiming=off  block_type=delay
      settings: infoedit=Hardware notes: A delay line is a chain, each link of which is an SRL16 followed by a flip-flop. If register retiming is enabled, the delay line is a chain of flip-flops.  block_version=8.2
  Display : Display
  Display1 : Display
  Display2 : Display
  Register : xbsIndex_r4/Register  init=0  rst=on  en=off  dbl_ovrd=off  block_type=register
      settings: block_version=8.2
  Register1 : xbsIndex_r4/Register  init=0  rst=off  en=off  dbl_ovrd=off  block_type=register
      settings: block_version=8.2
  Reinterpret : xbsIndex_r4/Reinterpret  force_arith_type=on  arith_type="Signed  (2's comp)"  force_bin_pt=on  bin_pt=0  block_type=cast
      settings: infoedit="Changes type of samples without altering their binary representation.<P><P>Hardware notes: In hardware this block costs nothing.<P><P>Example:  Suppose the input is 6 bits wide, signed, with 2 fractional bits, and the output is forced to unsigned with 0 fractional bits.  Then an input of -2.0 (1110.00 in binary 2's complement) becomes an output of 56 (111000 in binary)."  block_version=VER_STRING_GOES_HERE
  Reinterpret1 : xbsIndex_r4/Reinterpret  force_arith_type=on  arith_type="Signed  (2's comp)"  force_bin_pt=on  bin_pt=0  block_type=cast
      settings: infoedit="Changes type of samples without altering their binary representation.<P><P>Hardware notes: In hardware this block costs nothing.<P><P>Example:  Suppose the input is 6 bits wide, signed, with 2 fractional bits, and the output is forced to unsigned with 0 fractional bits.  Then an input of -2.0 (1110.00 in binary 2's complement) becomes an output of 56 (111000 in binary)."  block_version=VER_STRING_GOES_HERE
  Relational : xbsIndex_r4/Relational  mode=a=b  en=off  latency=1  dbl_ovrd=off  block_type=relational
      settings: block_version=8.2
  Terminator : Terminator
  Out : Outport
  wires:
  Count/1 -> ASR/2
  Data In/1 -> ASR/1
  ASR/1 -> Register1/1, Display2/1
  AddSub/1 -> Reinterpret/1, Display/1
  Coeff/1 -> Delay1/1
  Delay1/1 -> Reinterpret1/1, Display1/1
  PCIN/1 -> DSP48/3
  Register1/1 -> AddSub/1
  Symm Data/1 -> Delay3/1
  Count Inv/1 -> ASR1/2, Relational/1
  Delay3/1 -> ASR1/1
  ASR1/1 -> Register/1
  Constant/1 -> Relational/2
  Relational/1 -> Register/2
  Register/1 -> AddSub/2
  Reinterpret/1 -> DSP48/1
  Reinterpret1/1 -> DSP48/2
  Constant3/1 -> DSP48/4
  DSP48/1 -> Terminator/1
  DSP48/2 -> Out/1

== system Casc_Filter_reva/DDC/DDC A/Polyphase Kaiser FIR Filter/Q Accumulator ==
  Count : Inport
  Sum : Inport  Port=2
  Constant : xbsIndex_r4/Constant  arith_type=Signed (2's comp)  const=16383  n_bits=48  bin_pt=0  explicit_period=off  period=1  equ=P=C  opselect=C  inp2=PCIN>>17  opr=+  inp1=P  carry=CIN  dbl_ovrd=off  block_type=constant
      settings: block_version=8.2
  Constant1 : xbsIndex_r4/Constant  arith_type=Unsigned  const=0  n_bits=1  bin_pt=0  explicit_period=off  period=1  equ=P=C  opselect=C  inp2=PCIN>>17  opr=+  inp1=P  carry=CIN  dbl_ovrd=off  block_type=constant
      settings: block_version=8.2
  Constant6 : xbsIndex_r4/Constant  arith_type=Signed (2's comp)  const=0  n_bits=18  bin_pt=0  explicit_period=off  period=1  equ=P=PCIN+(A*B)  opselect=PCIN + A*B  inp2=PCIN>>17  opr=+  inp1=P  carry=CIN  dbl_ovrd=off  block_type=constant
      settings: block_version=8.2
  Constant7 : xbsIndex_r4/Constant  arith_type=Signed (2's comp)  const=0  n_bits=18  bin_pt=0  explicit_period=off  period=1  equ=P=PCIN+(A*B)  opselect=PCIN + A*B  inp2=PCIN>>17  opr=+  inp1=P  carry=CIN  dbl_ovrd=off  block_type=constant
      settings: block_version=8.2
  Constant8 : xbsIndex_r4/Constant  arith_type=DSP48 Instruction  const=1  n_bits=16  bin_pt=14  explicit_period=off  period=1  equ=P=PCIN+(P)  opselect=Custom  inp2=PCIN  opr=+  inp1=P  carry=0  dbl_ovrd=off  block_type=constant
      settings: block_version=8.2
  Constant9 : xbsIndex_r4/Constant  arith_type=DSP48 Instruction  const=1  n_bits=16  bin_pt=14  explicit_period=off  period=1  equ=P=PCIN+(C)  opselect=Custom  inp2=PCIN  opr=+  inp1=C  carry=0  dbl_ovrd=off  block_type=constant
      settings: block_version=8.2
  DSP2 : xbsIndex_r4/DSP48  use_b=Direct from B Port  use_op=on  use_creg=on  use_pcin=on  use_pcout=off  use_bcout=off  rst_all=off  en_all=off  pipeline_a=0  pipeline_b=0  pipeline_c=on  pipeline_p=on  pipeline_mult=off  pipeline_opmode=on  pipeline_sub=off  pipeline_carryin=off  pipeline_carryinsel=off  rst_a=off  rst_b=off  rst_c=off  rst_mult=off  rst_p=off  rst_carry_in=off  rst_ctrl=off  en_a=off  en_b=off  en_c=off  en_mult=off  en_p=off  en_carry_in=off  en_ctrl=off  dbl_ovrd=off  use_synth_model=off  xl_useadderonly=on  block_type=dsp48
      settings: block_version=8.2
  Delay : xbsIndex_r4/Delay  en=off  latency=2  dbl_ovrd=off  reg_retiming=off  block_type=delay
      settings: infoedit=Hardware notes: A delay line is a chain, each link of which is an SRL16 followed by a flip-flop. If register retiming is enabled, the delay line is a chain of flip-flops.  block_version=8.2
  Down Sample1 : xbsIndex_r4/Down Sample  sample_ratio=downsample  sample_phase="Last Value of Frame  (most efficient)"  en=off  latency=1  dbl_ovrd=off  block_type=dsamp
      settings: block_version=8.2
  Mux : xbsIndex_r4/Mux  inputs=2  en=off  latency=1  precision=Full  arith_type=Unsigned  n_bits=16  bin_pt=14  quantization=Truncate  overflow=Wrap  dbl_ovrd=off  block_type=mux
      settings: block_version=8.2
  Register : xbsIndex_r4/Register  init=0  rst=off  en=off  dbl_ovrd=off  block_type=register
      settings: block_version=8.2
  Register1 : xbsIndex_r4/Register  Orientation=down  init=0  rst=off  en=on  dbl_ovrd=off  block_type=register
      settings: block_version=8.2
  Reinterpret : xbsIndex_r4/Reinterpret  force_arith_type=on  arith_type="Signed  (2's comp)"  force_bin_pt=on  bin_pt=17  block_type=reinterpret
      settings: infoedit="Changes signal type without altering the binary representation.   You can changed the signal between signed and unsigned, and relocate the binary point.<P><P>Hardware notes: In hardware this block costs nothing.<P><P>Example:  Suppose the input is 6 bits wide, signed, with 2 fractional bits, and the output is forced to unsigned with 0 fractional bits.  Then an input of -2.0 (1110.00 in binary 2's complement) becomes an output of 56 (111000 in binary)."  block_version=8.2
  Relational : xbsIndex_r4/Relational  mode=a=b  en=off  latency=6  dbl_ovrd=off  block_type=relational
      settings: block_version=8.2
  Slice : xbsIndex_r4/Slice  nbits=16  boolean_output=off  mode=Two Bit Locations  bit1=-15  base1=MSB of Input  bit0=15  base0=LSB of Input  dbl_ovrd=off  block_type=slice
      settings: infoedit="Extracts a given range of bits from each input sample and presents it at the output.  The output type is ordinarily unsigned with binary point at zero, but can be Boolean when the slice is one bit wide.<P><P>Hardware notes: In hardware this block costs nothing."  block_version=8.2
  Out : Outport
  wires:
  Register1/1 -> Down Sample1/1
  Constant1/1 -> Relational/2
  Count/1 -> Relational/1
  Relational/1 -> Mux/1, Delay/1
  Reinterpret/1 -> Register/1
  Constant6/1 -> DSP2/1
  Constant7/1 -> DSP2/2
  DSP2/1 -> Register1/1
  Constant9/1 -> Mux/3
  Constant8/1 -> Mux/2
  Delay/1 -> Register1/2
  Slice/1 -> Reinterpret/1
  Register/1 -> Out/1
  Mux/1 -> DSP2/5
  Sum/1 -> DSP2/4
  Constant/1 -> DSP2/3
  Down Sample1/1 -> Slice/1
